simulink model "desktop_publish_subscribe"  (R2020a)
settings: Solver=FixedStepAuto  StartTime=0.0  StopTime=inf  RelTol=1e-3  EnableMultiTasking=on
PreLoadFcn:
  | Ts = 0.01;
model workspace (MAT data in the model file):
  SL_ROS_VariableLengthArrays_MaxSizes.CommonInfo.ArrayTruncateAction = 'EmitWarning'
  SL_ROS_VariableLengthArrays_MaxSizes.MsgTypeMap = containers.Map
  SL_ROS_VariableLengthArrays_MaxSizes.MsgTypeMap.serialization.keys = {'sensor_msgs/Image'}
  SL_ROS_VariableLengthArrays_MaxSizes.MsgTypeMap.serialization.values{1}(1).PropertyName = 'Data'
  SL_ROS_VariableLengthArrays_MaxSizes.MsgTypeMap.serialization.values{1}(1).DataType = 'uint8'
  SL_ROS_VariableLengthArrays_MaxSizes.MsgTypeMap.serialization.values{1}(1).MaxLength = 57600
  SL_ROS_VariableLengthArrays_MaxSizes.MsgTypeMap.serialization.values{1}(2).PropertyName = 'Encoding'
  SL_ROS_VariableLengthArrays_MaxSizes.MsgTypeMap.serialization.values{1}(2).DataType = 'uint8'
  SL_ROS_VariableLengthArrays_MaxSizes.MsgTypeMap.serialization.values{1}(2).MaxLength = 5
  SL_ROS_VariableLengthArrays_MaxSizes.MsgTypeMap.serialization.uniformity = 0
  SL_ROS_VariableLengthArrays_MaxSizes.MsgTypeMap.serialization.keyType = 'char'
  SL_ROS_VariableLengthArrays_MaxSizes.MsgTypeMap.serialization.valueType = 'any'
undefined symbols (not defined in the file): B, G, R
libraries: robotlib x6
settings Model: SimulationMode=external  Creator=The MathWorks, Inc.  LastModifiedBy=mmordeka
settings DataIOCC: SaveFormat=Array  ReturnWorkspaceOutputs=off
settings OptimizationCC: EnhancedBackFolding=on  PassReuseOutputArgsAs=Individual arguments  ZeroExternalMemoryAtStartup=off  ZeroInternalMemoryAtStartup=off  MaxStackSize=64  OptimizeBlockOrder=speed  DifferentSizesBufferReuse=on  OptimizationCustomize=off  EfficientTunableParamExpr=on
settings DebuggingCC: SolverPrmCheckMsg=warning  ParameterTunabilityLossMsg=error  AllowSymbolicDim=off  SFUnexpectedBacktrackingDiag=warning  SFNoUnconditionalDefaultTransitionDiag=warning  ArithmeticOperatorsInVariantConditions=warning
settings HardwareCC: ProdBitPerPointer=32  ProdBitPerSizeT=32  ProdBitPerPtrDiffT=32  ProdLargestAtomicInteger=Long  ProdLargestAtomicFloat=Double  ProdWordSize=32  ProdHWDeviceType=ARM Compatible->ARM Cortex
settings ModelReferenceCC: PropagateSignalLabelsOutOfModel=off
settings SFSimCC: SimUseLocalCustomCode=off  CustomCodeUndefinedFunction=UseInterfaceOnly
settings RTWCC: SystemTargetFile=ert.tlc  HardwareBoard=Raspberry Pi - Robot Operating System (ROS)  TemplateMakefile=ert_default_tmf  GenerateReport=on  RTWUseLocalCustomCode=off  Toolchain=Catkin  IncludeHyperlinkInReport=on  LaunchReport=on  TargetLang=C++  GenerateTraceInfo=on  GenerateTraceReport=on  GenerateTraceReportSl=on  GenerateTraceReportSf=on  GenerateTraceReportEml=on
settings CodeAppCC: ForceParamTrailComments=on  IgnoreCustomStorageClasses=off  OperatorAnnotations=on  SimulinkDataObjDesc=on  SFDataObjDesc=on  InsertBlockDesc=on
settings ERTTargetCC: ExtMode=on
settings ConfigComp: CovMetricSettings=dw  CovHtmlReporting=on  CovSaveCumulativeToWorkspaceVar=on  CovSaveSingleToWorkspaceVar=on  CovExternalEMLEnable=off  CovSFcnEnable=off

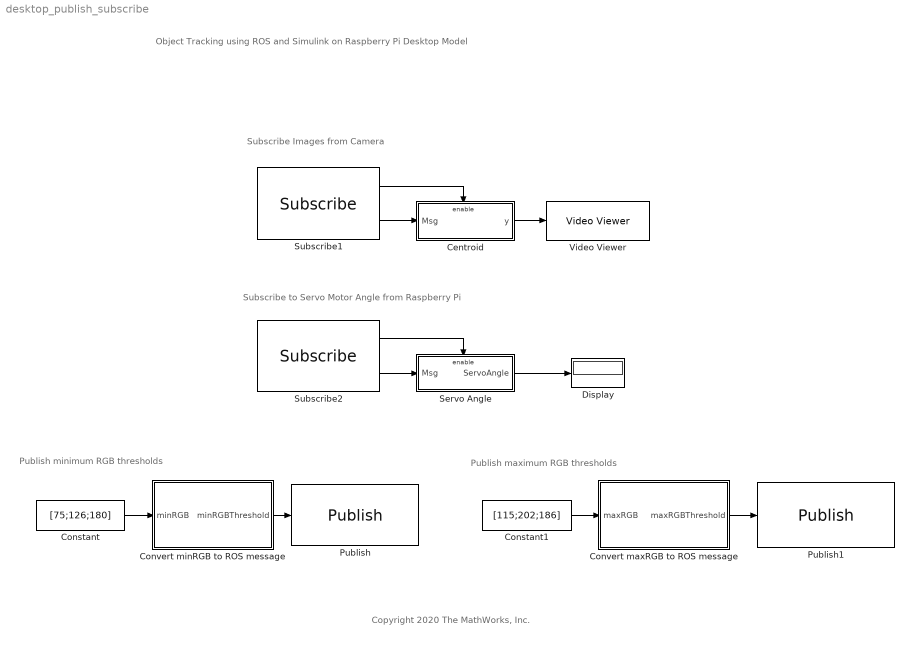
== system desktop_publish_subscribe ==
  note: Publish maximum RGB thresholds
  note: Publish minimum RGB thresholds
  note: Subscribe to Servo Motor Angle from Raspberry Pi
  note: Subscribe Images from Camera
  note: Object Tracking using ROS and Simulink on Raspberry Pi
      | Desktop Model
  note: Copyright 2020 The MathWorks, Inc.
  Centroid : Subsystem
  Constant : Constant  Value=[75;126;180]  OutDataTypeStr=Inherit: Inherit via back propagation  SampleTime=Ts
  Constant1 : Constant  Value=[115;202;186]  OutDataTypeStr=Inherit: Inherit via back propagation  SampleTime=Ts
  Convert maxRGB to ROS message : Subsystem
  Convert minRGB to ROS message : Subsystem
  Display : Display
  Publish : robotlib/Publish  topicSource=Specify your own  topic=/minRGBThreshold  messageType=std_msgs/ColorRGBA  messageQueueLength=1
  Publish1 : robotlib/Publish  topicSource=Specify your own  topic=/maxRGBThreshold  messageType=std_msgs/ColorRGBA  messageQueueLength=1
  Servo Angle : Subsystem
  Subscribe1 : robotlib/Subscribe  topicSource=Specify your own  topic=/camera  messageType=sensor_msgs/Image  sampleTime=Ts  messageQueueLength=51
  Subscribe2 : robotlib/Subscribe  topicSource=Specify your own  topic=/servo_angle  messageType=std_msgs/UInt8  sampleTime=Ts  messageQueueLength=51
  Video Viewer : VideoViewer  FigPos=[385 571 418 304]
  wires:
  Subscribe1/1 -> Centroid/Enable
  Subscribe1/2 -> Centroid/1(Msg)
  Servo Angle/1(ServoAngle) -> Display/1
  Subscribe2/1 -> Servo Angle/Enable
  Subscribe2/2 -> Servo Angle/1(Msg)
  Constant/1 -> Convert minRGB to ROS message/1(minRGB)
  Convert minRGB to ROS message/1(minRGBThreshold) -> Publish/1
  Constant1/1 -> Convert maxRGB to ROS message/1(maxRGB)
  Convert maxRGB to ROS message/1(maxRGBThreshold) -> Publish1/1
  Centroid/1(y) -> Video Viewer/1

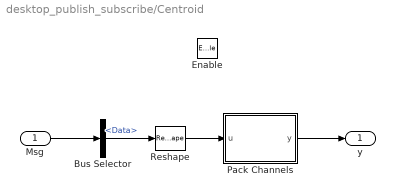
== system desktop_publish_subscribe/Centroid ==
  Msg : Inport
  Enable : EnablePort
  Bus Selector : BusSelector  OutputSignals=Data
  Pack Channels : MATLAB Function  TreatAsAtomicUnit=on
  Reshape : Reshape  OutputDimensionality=Customize  OutputDimensions=[160 120 3]
  y : Outport
  wires:
  Msg/1 -> Bus Selector/1
  Bus Selector/1 -> Reshape/1  "<Data>"
  Reshape/1 -> Pack Channels/1(u)
  Pack Channels/1(y) -> y/1

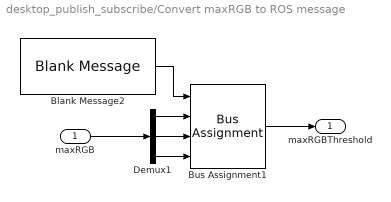
== system desktop_publish_subscribe/Convert maxRGB to ROS message ==
  maxRGB : Inport
  Blank Message2 : robotlib/Blank Message  messageClass=Message  entityType=std_msgs/ColorRGBA  messageType=std_msgs/ColorRGBA  SampleTime=Ts
  Bus Assignment1 : BusAssignment  AssignedSignals=R,G,B
  Demux1 : Demux  Outputs=3
  maxRGBThreshold : Outport
  wires:
  Blank Message2/1 -> Bus Assignment1/1
  maxRGB/1 -> Demux1/1
  Demux1/2 -> Bus Assignment1/3
  Bus Assignment1/1 -> maxRGBThreshold/1
  Demux1/3 -> Bus Assignment1/4
  Demux1/1 -> Bus Assignment1/2

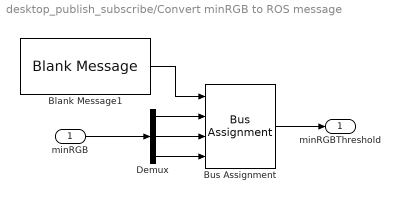
== system desktop_publish_subscribe/Convert minRGB to ROS message ==
  minRGB : Inport
  Blank Message1 : robotlib/Blank Message  messageClass=Message  entityType=std_msgs/ColorRGBA  messageType=std_msgs/ColorRGBA  SampleTime=Ts
  Bus Assignment : BusAssignment  AssignedSignals=R,G,B
  Demux : Demux  Outputs=3
  minRGBThreshold : Outport
  wires:
  Demux/1 -> Bus Assignment/2
  Demux/2 -> Bus Assignment/3
  Demux/3 -> Bus Assignment/4
  Blank Message1/1 -> Bus Assignment/1
  Bus Assignment/1 -> minRGBThreshold/1
  minRGB/1 -> Demux/1

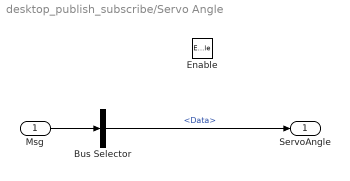
== system desktop_publish_subscribe/Servo Angle ==
  Msg : Inport
  Enable : EnablePort
  Bus Selector : BusSelector  OutputSignals=Data
  ServoAngle : Outport
  wires:
  Bus Selector/1 -> ServoAngle/1  "<Data>"
  Msg/1 -> Bus Selector/1

== matlab function desktop_publish_subscribe/Centroid/Pack Channels ==
  data: u input; y output
function y = fcn(u)

R = u(:,:,1)';
G = u(:,:,2)';
B = u(:,:,3)';

y = cat(3,R,G,B);
